simulink model "CiEngineCore"  (R2020a)
settings: Solver=VariableStepAuto  StartTime=0.0  StopTime=inf  RelTol=1e-3  EnableMultiTasking=on
model workspace (MAT data in the model file):
  AirFilterArea = 0.000962112750162
  AirIntakeVol = 0.0018
  C_eng = 40000
  CompEff = [0.2 0.2 0.2 0.2 0.2 0.2 0.2 0.2 0.2 0.2 0.2 0.2 ... (6000 elements, 60x100)]
  CompMassFlwRate = [0 0.00256701884694 0.00511455880808 0.00766649491749 0.0102195028494 0.0127729401774 0.0153265889731 0.017880362476 0.0204342099213 0.0229881081418 0.0255420430633 0.0280960028754 ... (6000 elements, 60x100)]
  CompPrsRatioBreakPoints = [1 1.02808080808 1.05616161616 1.08424242424 1.11232323232 1.1404040404 1.16848484848 1.19656565657 1.22464646465 1.25272727273 1.28080808081 1.30888888889 1.33696969697 1.36505050505 1.39313131313 1.42121212121 1.44929292929 1.47737373737 1.50545454545 1.53353535354 1.56161616162 1.5896969697 1.61777777778 1.64585858586 1.67393939394 1.70202020202 1.7301010101 1.75818181818 1.78626262626 1.81434343434 1.84242424242 1.87050505051 1.89858585859 1.92666666667 1.95474747475 1.98282828283 2.01090909091 2.03898989899 2.06707070707 2.09515151515 2.12323232323 2.15131313131 2.17939393939 2.20747474747 2.23555555556 2.26363636364 2.29171717172 2.3197979798 2.34787878788 2.37595959596 2.40404040404 2.43212121212 2.4602020202 2.48828282828 2.51636363636 2.54444444444 2.57252525253 2.60060606061 2.62868686869 2.65676767677 2.68484848485 2.71292929293 2.74101010101 2.76909090909 2.79717171717 2.82525252525 2.85333333333 2.88141414141 2.90949494949 2.93757575758 2.96565656566 2.99373737374 3.02181818182 3.0498989899 3.07797979798 3.10606060606 3.13414141414 3.16222222222 3.1903030303 3.21838383838 3.24646464646 3.27454545455 3.30262626263 3.33070707071 3.35878787879 3.38686868687 3.41494949495 3.44303030303 3.47111111111 3.49919191919 3.52727272727 3.55535353535 3.58343434343 3.61151515152 3.6395959596 3.66767676768 3.69575757576 3.72383838384 3.75191919192 3.78]
  CompRefPrs = 101325
  CompRefTemp = 300
  CompSpdBreakPoints = [0 422.344846438 844.689692876 1267.03447648 1689.3794067 2111.72412747 2534.06895296 2956.4139879 3378.75881339 3801.10374361 4223.44825494 4645.79349931 5068.13790593 5490.48294086 5912.8279758 6335.17238241 6757.51762678 7179.86182396 7602.20748721 8024.55231271 8446.89650988 8869.24133538 9291.58699863 9713.9311958 10136.2759166 10558.6216845 10980.9658817 11403.3100789 11825.6558469 12248.0005676 12670.3447648 13092.6904281 13515.0352536 13937.3794507 14359.7246951 14782.0688923 15204.4151839 15626.759381 16049.1046254 16471.4488226 16893.7930198 17316.1382641 17738.4824613 18160.8287529 18583.1729501 19005.5181944 19427.8623916 19850.207636 20272.5518332 20694.8981247 21117.2423219 21539.5865191 21961.9317635 22384.2770078 22806.621205 23228.9654022 23651.3116937 24073.6558909 24496.0011353 24918.3453325]
  CoolantTemp = 310
  Cps = 2
  EgrArea = 0.000314159265359
  EgrCoolantTemp = 360
  EgrEffectiveness = 0.8
  ExhSysArea = 0.000804247719319
  ExhSysVol = 0.0008
  IcEffectiveness = 0.9
  LHV = 47300000
  NCyl = 4
  Pstd = 101325
  Rair = 287.05
  Rexh = 297
  Sinj = 6.45161290323
  T_cool_start = 355
  T_coolnt_init = 355
  T_coolnt_max = 375
  Tstd = 293.15
  TurbEff = [0.008 0.008 0.008 0.008 0.008 0.008 0.008 0.008 0.008 0.008 0.008 0.008 ... (28800 elements, 60x80x6)]
  TurbMassFlwRate = [0 0 0 0 0 0 0 0 0 0 0 0 ... (28800 elements, 60x80x6)]
  TurbPrsRatioBreakPoints = [1 1.03481012658 1.06962025316 1.10443037975 1.13924050633 1.17405063291 1.20886075949 1.24367088608 1.27848101266 1.31329113924 1.34810126582 1.38291139241 1.41772151899 1.45253164557 1.48734177215 1.52215189873 1.55696202532 1.5917721519 1.62658227848 1.66139240506 1.69620253165 1.73101265823 1.76582278481 1.80063291139 1.83544303797 1.87025316456 1.90506329114 1.93987341772 1.9746835443 2.00949367089 2.04430379747 2.07911392405 2.11392405063 2.14873417722 2.1835443038 2.21835443038 2.25316455696 2.28797468354 2.32278481013 2.35759493671 2.39240506329 2.42721518987 2.46202531646 2.49683544304 2.53164556962 2.5664556962 2.60126582278 2.63607594937 2.67088607595 2.70569620253 2.74050632911 2.7753164557 2.81012658228 2.84493670886 2.87974683544 2.91455696203 2.94936708861 2.98417721519 3.01898734177 3.05379746835 3.08860759494 3.12341772152 3.1582278481 3.19303797468 3.22784810127 3.26265822785 3.29746835443 3.33227848101 3.36708860759 3.40189873418 3.43670886076 3.47151898734 3.50632911392 3.54113924051 3.57594936709 3.61075949367 3.64556962025 3.68037974684 3.71518987342 3.75]
  TurbRackBreakPoints = [0 0.2 0.3 0.5 0.7 1]
  TurbRefPrs = 101325
  TurbRefTemp = 300
  TurbSpdBreakPoints = [0 267.361773363 534.723546727 802.08532009 1069.44709345 1336.80886682 1604.17064018 1871.53241354 2138.89418691 2406.25596027 2673.61773363 2940.979507 3208.34128036 3475.70305372 3743.06482709 4010.42660045 4277.78837381 4545.15014718 4812.51192054 5079.8736939 5347.23546727 5614.59724063 5881.95901399 6149.32078736 6416.68256072 6684.04433408 6951.40610745 7218.76788081 7486.12965417 7753.49142754 8020.8532009 8288.21497426 8555.57674763 8822.93852099 9090.30029435 9357.66206772 9625.02384108 9892.38561444 10159.7473878 10427.1091612 10694.4709345 10961.8327079 11229.1944813 11496.5562546 11763.918028 12031.2798014 12298.6415747 12566.0033481 12833.3651214 13100.7268948 13368.0886682 13635.4504415 13902.8122149 14170.1739883 14437.5357616 14704.897535 14972.2593083 15239.6210817 15506.9828551 15774.3446284]
  TurboInertia = 6e-06
  Vd = 0.0015
  Vexh = 0.000696349540849
  Vint = 0.00286
  afr_stoich = 14.6
  cp_air = 1005
  cp_exh = 1005
  f_co = [1.40212981041e-06 1.40212981041e-06 1.6332261526e-06 1.85316257772e-06 2.13933731744e-06 2.5578774362e-06 3.5801963158e-06 5.71066968323e-06 9.06691784867e-06 1.17856264254e-05 1.13266430068e-05 1.17075290539e-05 ... (240 elements, 16x15)]
  f_co2 = [0.0565058276487 0.0565058276487 0.0680775298139 0.0795416117649 0.0927502758383 0.108898516704 0.135970777083 0.163224038089 0.18390566243 0.187824483941 0.180854201863 0.181624048607 ... (240 elements, 16x15)]
  f_exhfrac_n_bpt = [750 1053.57142857 1357.14285714 1660.71428571 1964.28571429 2267.85714286 2571.42857143 2875 3178.57142857 3482.14285714 3785.71428571 4089.28571429 4392.85714286 4696.42857143 5000]
  f_exhfrac_trq_bpt = [0 15 26.4285714286 37.8571428571 49.2857142857 60.7142857143 72.1428571429 83.5714285714 95 106.428571429 117.857142857 129.285714286 140.714285714 152.142857143 163.571428571 175]
  f_fric_temp_bpt = [274 276 278 280 282 284 286 288 290 292 294 296 298 300 302 304 306 308 310 312 314 316 318 320 322 324 326 328 330 332 334 336 338 340 342 344 346 348 350 352 354 356 358 360 362 364 366 368 370 372 374 376 378 380]
  f_fric_temp_mod = [3.96 3.22 2.56 2.26 2.11 2 1.9 1.83 1.76 1.7 1.65 1.6 1.55 1.49 1.44 1.41 1.38 1.35 1.32 1.3 1.27 1.25 1.24 1.21 1.2 1.18 1.16 1.15 1.13 1.12 1.11 1.1 1.09 1.08 1.07 1.06 1.05 1.05 1.04 1.03 1.02 1.02 1.01 1.01 1 1 1 0.999 0.997 0.995 0.993 0.991 0.989 0.987]
  f_hc = [1.08896576916e-07 1.08896576916e-07 1.53414498342e-07 2.00715453959e-07 2.48790869997e-07 2.97869368014e-07 3.52504999231e-07 4.04349945817e-07 4.52780325277e-07 4.91342452993e-07 4.91996758973e-07 4.96487624267e-07 ... (240 elements, 16x15)]
  f_nox = [9.38886565825e-05 9.38886565825e-05 0.000158278744526 0.000381657424268 0.00062836202089 0.000865097048745 0.000965103000667 0.00083216127124 0.00082959112316 0.00143554359074 0.00196340813932 0.0020351396325 ... (240 elements, 16x15)]
  f_nv = [0.954646224834 0.927678310575 0.901063682417 0.875710037198 0.852450535311 0.831986822876 0.814844392337 0.80134438932 0.791593989181 0.785495277781 0.782770492696 0.782999798686 ... (450 elements, 30x15)]
  f_nv_n_bpt = [1000 1285.71428571 1571.42857143 1857.14285714 2142.85714286 2428.57142857 2714.28571429 3000 3285.71428571 3571.42857143 3857.14285714 4142.85714286 4428.57142857 4714.28571429 5000]
  f_nv_prs_bpt = [95 100.344827586 105.689655172 111.034482759 116.379310345 121.724137931 127.068965517 132.413793103 137.75862069 143.103448276 148.448275862 153.793103448 159.137931034 164.482758621 169.827586207 175.172413793 180.517241379 185.862068966 191.206896552 196.551724138 201.896551724 207.24137931 212.586206897 217.931034483 223.275862069 228.620689655 233.965517241 239.310344828 244.655172414 250]
  f_t_exh = [358.711368346 429.963145924 497.987869771 559.016510887 625.497016294 690.207854611 731.780908025 749.899407528 764.155922317 789.797182974 824.513264157 858.92580636 ... (240 elements, 16x15)]
  f_t_exh_f_bpt = [0 3.57 6.855 10.14 13.425 16.71 19.995 23.28 26.565 29.85 33.135 36.42 39.705 42.99 46.275 49.56]
  f_t_exh_n_bpt = [1000 1285.71428571 1571.42857143 1857.14285714 2142.85714286 2428.57142857 2714.28571429 3000 3285.71428571 3571.42857143 3857.14285714 4142.85714286 4428.57142857 4714.28571429 5000]
  f_tq_nf = [0 4.01032735147 17.4541547029 30.8399626872 43.6894710619 54.6724182266 65.9817429981 74.8844587697 82.0625281792 91.0474591726 100.604737295 107.761633858 ... (320 elements, 20x16)]
  f_tq_nf_f_bpt = [0 2.63157894737 5.26315789474 7.89473684211 10.5263157895 13.1578947368 15.7894736842 18.4210526316 21.0526315789 23.6842105263 26.3157894737 28.9473684211 31.5789473684 34.2105263158 36.8421052632 39.4736842105 42.1052631579 44.7368421053 47.3684210526 50]
  f_tq_nf_n_bpt = [0 1000 1285.71428571 1571.42857143 1857.14285714 2142.85714286 2428.57142857 2714.28571429 3000 3285.71428571 3571.42857143 3857.14285714 4142.85714286 4428.57142857 4714.28571429 5000]
  f_tqs_emap = [101325 101325 101325 101325 101325 101325 101325 101325 101325 101325 101325 101325 ... (240 elements, 15x16)]
  f_tqs_exht = [293.15 293.15 293.15 293.15 293.15 293.15 293.15 293.15 293.15 293.15 293.15 293.15 ... (240 elements, 15x16)]
  f_tqs_exht_fuelpress_eff = [1  1  1  1  1  1  1  1  1  1  1  1  1  1  1  1; 1  1  1  1  1  1  1  1  1  1  1  1  1  1  1  1; 1  1  1  1  1  1  1  1  1  1  1  1  1  1  1  1; 1  1  1  1  1  1  1  1  1  1  1  1  1  1  1  1; 1  1  1  1  1  1  1  1  1  1  1  1  1  1  1  1; 1  1  1  1  1  1  1  1  1  1  1  1  1  1  1  1; 1  1  1  1  1  1  1  1  1  1  1  1  1  1  1  1; 1  1  1  1  1  1  1  1  1  1  1  1  1  1  1  1; 1  1  1  1  1  1  1  1  1  1  1  1  1  1  1  1; 1  1  1  1  1  1  1  1  1  1  1  1  1  1  1  1; 1  1  1  1  1  1  1  1  1  1  1  1  1  1  1  1; 1  1  1  1  1  1  1  1  1  1  1  1  1  1  1  1; 1  1  1  1  1  1  1  1  1  1  1  1  1  1  1  1; 1  1  1  1  1  1  1  1  1  1  1  1  1  1  1  1; 1  1  1  1  1  1  1  1  1  1  1  1  1  1  1  1]
  f_tqs_exht_mainsoi_eff = [1 1 1 1 1 1 1 1 1 1 1 1 ... (240 elements, 15x16)]
  f_tqs_exht_map_eff = [1.11693337379 1.10383565741 1.07527138779 1.03804427558 1 0.975297725101 0.950398019177 0.924393698482 0.899021655666 0.876045599233 0.858573316119 0.844444824038 ... (225 elements, 15x15)]
  f_tqs_exht_mat_eff = [1 1 1 1 1 1 1 1 1 1 1 1 ... (240 elements, 15x16)]
  f_tqs_exht_o2pct_eff = [1 1 1 1 1 1 1 1 1 1 1 1 ... (240 elements, 15x16)]
  f_tqs_exht_post_inj_wall_htc = 0
  f_tqs_f_bpt = [0; 3.57142857143; 7.14285714286; 10.7142857143; 14.2857142857; 17.8571428571; 21.4285714286; 25; 28.5714285714; 32.1428571429; 35.7142857143; 39.2857142857; 42.8571428571; 46.4285714286; 50]
  f_tqs_f_burned_soi_limit = 500
  f_tqs_f_inj_type = 0
  f_tqs_f_post_sum_bpt = [0 3.57142857143 7.14285714286 10.7142857143 14.2857142857 17.8571428571 21.4285714286 25 28.5714285714 32.1428571429 35.7142857143 39.2857142857 42.8571428571 46.4285714286 50]
  f_tqs_fmep = [0 0 0 0 0 0 0 0 0 0 0 0 ... (240 elements, 15x16)]
  f_tqs_fric_temp_bpt = [273.15; 275.166037736; 277.182075472; 279.198113208; 281.214150943; 283.230188679; 285.246226415; 287.262264151; 289.278301887; 291.294339623; 293.310377358; 295.326415094; 297.34245283; 299.358490566; 301.374528302; 303.390566038; 305.406603774; 307.422641509; 309.438679245; 311.454716981; 313.470754717; 315.486792453; 317.502830189; 319.518867925; 321.53490566; 323.550943396; 325.566981132; 327.583018868; 329.599056604; 331.61509434; 333.631132075; 335.647169811; 337.663207547; 339.679245283; 341.695283019; 343.711320755; 345.727358491; 347.743396226; 349.759433962; 351.775471698; 353.791509434; 355.80754717; 357.823584906; 359.839622642; 361.855660377; 363.871698113; 365.887735849; 367.903773585; 369.919811321; 371.935849057; 373.951886792; 375.967924528; 377.983962264; 380]
  f_tqs_fric_temp_mod = [1 1 1 1 1 1 1 1 1 1 1 1 ... (864 elements, 54x16)]
  f_tqs_fuelpress = [100  100  100  100  100  100  100  100  100  100  100  100  100  100  100  100; 100  100  100  100  100  100  100  100  100  100  100  100  100  100  100  100; 100  100  100  100  100  100  100  100  100  100  100  100  100  100  100  100; 100  100  100  100  100  100  100  100  100  100  100  100  100  100  100  100; 100  100  100  100  100  100  100  100  100  100  100  100  100  100  100  100; 100  100  100  100  100  100  100  100  100  100  100  100  100  100  100  100; 100  100  100  100  100  100  100  100  100  100  100  100  100  100  100  100; 100  100  100  100  100  100  100  100  100  100  100  100  100  100  100  100; 100  100  100  100  100  100  100  100  100  100  100  100  100  100  100  100; 100  100  100  100  100  100  100  100  100  100  100  100  100  100  100  100; 100  100  100  100  100  100  100  100  100  100  100  100  100  100  100  100; 100  100  100  100  100  100  100  100  100  100  100  100  100  100  100  100; 100  100  100  100  100  100  100  100  100  100  100  100  100  100  100  100; 100  100  100  100  100  100  100  100  100  100  100  100  100  100  100  100; 100  100  100  100  100  100  100  100  100  100  100  100  100  100  100  100]
  f_tqs_fuelpress_delta_bpt = [-30; -25.7142857143; -21.4285714286; -17.1428571429; -12.8571428571; -8.57142857143; -4.28571428571; 0; 4.28571428571; 8.57142857143; 12.8571428571; 17.1428571429; 21.4285714286; 25.7142857143; 30]
  f_tqs_fuelpress_eff = [1  1  1  1  1  1  1  1  1  1  1  1  1  1  1  1; 1  1  1  1  1  1  1  1  1  1  1  1  1  1  1  1; 1  1  1  1  1  1  1  1  1  1  1  1  1  1  1  1; 1  1  1  1  1  1  1  1  1  1  1  1  1  1  1  1; 1  1  1  1  1  1  1  1  1  1  1  1  1  1  1  1; 1  1  1  1  1  1  1  1  1  1  1  1  1  1  1  1; 1  1  1  1  1  1  1  1  1  1  1  1  1  1  1  1; 1  1  1  1  1  1  1  1  1  1  1  1  1  1  1  1; 1  1  1  1  1  1  1  1  1  1  1  1  1  1  1  1; 1  1  1  1  1  1  1  1  1  1  1  1  1  1  1  1; 1  1  1  1  1  1  1  1  1  1  1  1  1  1  1  1; 1  1  1  1  1  1  1  1  1  1  1  1  1  1  1  1; 1  1  1  1  1  1  1  1  1  1  1  1  1  1  1  1; 1  1  1  1  1  1  1  1  1  1  1  1  1  1  1  1; 1  1  1  1  1  1  1  1  1  1  1  1  1  1  1  1]
  f_tqs_imep_post_corr = [0  0  0  0  0  0  0  0  0  0  0  0  0  0  0; 0  0  0  0  0  0  0  0  0  0  0  0  0  0  0; 0  0  0  0  0  0  0  0  0  0  0  0  0  0  0; 0  0  0  0  0  0  0  0  0  0  0  0  0  0  0; 0  0  0  0  0  0  0  0  0  0  0  0  0  0  0; 0  0  0  0  0  0  0  0  0  0  0  0  0  0  0; 0  0  0  0  0  0  0  0  0  0  0  0  0  0  0; 0  0  0  0  0  0  0  0  0  0  0  0  0  0  0; 0  0  0  0  0  0  0  0  0  0  0  0  0  0  0; 0  0  0  0  0  0  0  0  0  0  0  0  0  0  0; 0  0  0  0  0  0  0  0  0  0  0  0  0  0  0; 0  0  0  0  0  0  0  0  0  0  0  0  0  0  0; 0  0  0  0  0  0  0  0  0  0  0  0  0  0  0; 0  0  0  0  0  0  0  0  0  0  0  0  0  0  0; 0  0  0  0  0  0  0  0  0  0  0  0  0  0  0]
  f_tqs_imepg = [0 158686.534722 343074.265588 507983.203346 653190.552872 792520.266872 898623.174707 1024926.34814 1192408.65419 1362289.29874 1538616.81914 1722468.1753 ... (240 elements, 15x16)]
  f_tqs_lambda_bpt = [1.5 1.67857142857 1.85714285714 2.03571428571 2.21428571429 2.39285714286 2.57142857143 2.75 2.92857142857 3.10714285714 3.28571428571 3.46428571429 3.64285714286 3.82142857143 4]
  f_tqs_mainsoi = [-5.65203706782 -5.56485950617 -5.32737749535 -4.90693102774 -4.39157989496 -2.6685350622 -1.13269707429 -0.442811837066 0.0846384555918 0.793458776955 1.62426195607 2.45698560821 ... (240 elements, 15x16)]
  f_tqs_mainsoi_delta_bpt = [-15; -12.8571428571; -10.7142857143; -8.57142857143; -6.42857142857; -4.28571428571; -2.14285714286; 0; 2.14285714286; 4.28571428571; 6.42857142857; 8.57142857143; 10.7142857143; 12.8571428571; 15]
  f_tqs_mainsoi_eff = [1 1 1 1 1 1 1 1 1 1 1 1 ... (240 elements, 15x16)]
  f_tqs_map = [101325 101325 101325 101325 101325 101325 101325 101325 101325 101325 101325 101325 ... (240 elements, 15x16)]
  f_tqs_map_eff = [0.876486797315 0.914614445767 0.94792295911 0.975703338034 1 1.02743787204 1.05216674291 1.07395048632 1.09371107566 1.11066007626 1.12521245816 1.14202789912 ... (225 elements, 15x15)]
  f_tqs_map_ratio_bpt = [0.8; 0.85; 0.9; 0.95; 1; 1.05; 1.1; 1.15; 1.2; 1.25; 1.3; 1.35; 1.4; 1.45; 1.5]
  f_tqs_mat = [293.15 293.15 293.15 293.15 293.15 293.15 293.15 293.15 293.15 293.15 293.15 293.15 ... (240 elements, 15x16)]
  f_tqs_mat_delta_bpt = [-55; -50; -45; -40; -35; -30; -25; -20; -15; -10; -5; 0; 5; 10; 15]
  f_tqs_mat_eff = [1 1 1 1 1 1 1 1 1 1 1 1 ... (240 elements, 15x16)]
  f_tqs_n_bpt = [0 500 750 1000 1250 1500 1750 2000 2250 2500 2750 3000 3250 3500 3750 4000]
  f_tqs_o2pct = [18.6138636402 19.5619833676 20.7378306586 22.1536730517 23.4120452691 23.8418651452 23.8693762547 23.8866954757 24.0193105899 24.2672589018 24.5893674985 24.9537951111 ... (240 elements, 15x16)]
  f_tqs_o2pct_delta_bpt = [-2; -1.33333333333; -0.666666666667; 0; 0.666666666667; 1.33333333333; 2; 2.66666666667; 3.33333333333; 4; 4.66666666667; 5.33333333333; 6; 6.66666666667; 7.33333333333]
  f_tqs_o2pct_eff = [1 1 1 1 1 1 1 1 1 1 1 1 ... (240 elements, 15x16)]
  f_tqs_pmep = [0 0 0 0 0 0 0 0 0 0 0 0 ... (240 elements, 15x16)]
  f_tqs_soi_post_cent_bpt = [150 160.714285714 171.428571429 182.142857143 192.857142857 203.571428571 214.285714286 225 235.714285714 246.428571429 257.142857143 267.857142857 278.571428571 289.285714286 300]
  fuel_lhv = 42000000
  tau_cool = 3000
undefined symbols (not defined in the file or in its folder): ThrAngToC
libraries: autolibfundflw x11, autolibboost x3, autolibcoreeng x1, simulink x1
(part 1 of 2)
settings Model: ModifiedByFormat=The MathWorks, Inc.  OrderedModelArguments=off  Creator=The MathWorks, Inc.  LastModifiedBy=The MathWorks, Inc.
settings SolverCC: DecoupledContinuousIntegration=on
settings DataIOCC: DSMLogging=off  ReturnWorkspaceOutputs=off
settings DebuggingCC: PregeneratedLibrarySubsystemCodeDiagnostic=none  ArithmeticOperatorsInVariantConditions=warning
settings SFSimCC: SimUseLocalCustomCode=off  CustomCodeUndefinedFunction=UseInterfaceOnly
settings RTWCC: RTWUseLocalCustomCode=off
settings CodeAppCC: StateflowObjectComments=on
settings GRTTargetCC: TargetLangStandard=C89/C90 (ANSI)
settings ConfigComp: CovMetricSettings=dsw  CovHtmlReporting=on  CovSaveCumulativeToWorkspaceVar=on  CovSaveSingleToWorkspaceVar=on  CovShowResultsExplorer=off  CovExternalEMLEnable=off
settings SimscapeCC: SimscapeNormalizeSystem=off  SimscapeNominalValues={1, 'bar'; 1, 'cm^3/s'; 1, 'bar*kg/s'; 1, 'kJ/kg'; 1, 'kW'; }

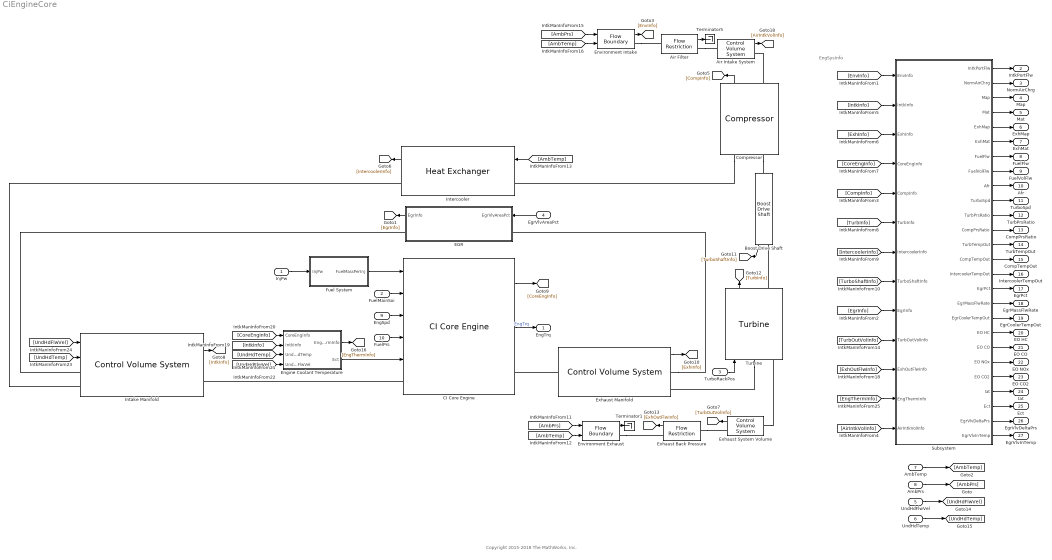
== system CiEngineCore ==
  note: EngSysInfo
  note: Copyright 2015-2018 The MathWorks, Inc.
  InjPw : Inport
  FuelMainSoi : Inport  Port=2
  TurboRackPos : Inport  Port=3
  EgrVlvAreaPct : Inport  Port=4
  UndHdFlwVel : Inport  Port=5
  UndHdTemp : Inport  Port=6
  AmbTemp : Inport  Port=7
  AmbPrs : Inport  Port=8
  EngSpd : Inport  Port=9
  FuelPrs : Inport  Port=10
  Air Filter : autolibfundflw/Flow Restriction  AreaPopup=Constant  ImageTypePopup=Cold  gamma=cp_air/(cp_air-Rair)  R=Rair  Plim=0.99  Aorf_cnst=AirFilterArea  Cd_cnst=1  Cd_ext=1  Dthr=50  ThrCd=[0.001; 0.735]  ThrAngBpts=[0; 90]
      settings: SourceProductBaseCode=PW
  Air Intake System : autolibfundflw/Control Volume System  NumInletPorts=1  NumOutletPorts=1  HeatTransferModelPopup=Constant  ImageTypePopup=Cold  Vch=AirIntakeVol  Pinit=101325  Tinit=298  R=Rair  cp=cp_air  q_he=0  ext_tbl=[40 160 740 2000]  ext_bpts=linspace(0,180,4)  Aext_conv=0.125  m_wall=7  cp_wall=900  Tmass=293.15  Dext_cond=0.004  Aext_cond=0.003  kext=25  Dint_cond=0.004  Aint_cond=0.003  kint=25  int_tbl=[40 160 740 2000]  int_bpts=linspace(0.0020,0.1100,4)  Aint_conv=0.125
      settings: SourceProductBaseCode=PW
  Boost Drive Shaft : autolibboost/Boost Drive Shaft  ShaftConfigPopup=Turbocharger  AddTrqTypePopup=No external torque  J_shaft=TurboInertia  w_0=0.0001  w_min=0.0001  w_max=1e6  eta_mech=1
      settings: SourceProductBaseCode=PW
  CI Core Engine : autolibcoreeng/CI Core Engine  TrqOptionPopup=Torque Structure  NCyl=NCyl  Tstd=Tstd  Cps=Cps  Vd=Vd  Rair=Rair  Pstd=Pstd  f_nv=f_nv  f_nv_prs_bpt=f_nv_prs_bpt  f_nv_n_bpt=f_nv_n_bpt  f_tq_nf=f_tq_nf  f_tq_nf_f_bpt=f_tq_nf_f_bpt  f_tq_nf_n_bpt=f_tq_nf_n_bpt  f_tqs_f_bpt=f_tqs_f_bpt  f_tqs_n_bpt=f_tqs_n_bpt  f_tqs_mainsoi=f_tqs_mainsoi  f_tqs_map=f_tqs_map  f_tqs_emap=f_tqs_emap  f_tqs_mat=f_tqs_mat  f_tqs_o2pct=f_tqs_o2pct  f_tqs_fuelpress=f_tqs_fuelpress  f_tqs_imepg=f_tqs_imepg  f_tqs_fmep=f_tqs_fmep  f_tqs_pmep=f_tqs_pmep  f_tqs_fric_temp_mod=f_tqs_fric_temp_mod  f_tqs_fric_temp_bpt=f_tqs_fric_temp_bpt  f_tqs_mainsoi_eff=f_tqs_mainsoi_eff  f_tqs_mainsoi_delta_bpt=f_tqs_mainsoi_delta_bpt  f_tqs_map_eff=f_tqs_map_eff  f_tqs_map_ratio_bpt=f_tqs_map_ratio_bpt  f_tqs_lambda_bpt=f_tqs_lambda_bpt  f_tqs_mat_eff=f_tqs_mat_eff  f_tqs_mat_delta_bpt=f_tqs_mat_delta_bpt  f_tqs_o2pct_eff=f_tqs_o2pct_eff  f_tqs_o2pct_delta_bpt=f_tqs_o2pct_delta_bpt  f_tqs_fuelpress_eff=f_tqs_fuelpress_eff  f_tqs_fuelpress_delta_bpt=f_tqs_fuelpress_delta_bpt  f_tqs_f_inj_type=f_tqs_f_inj_type  f_tqs_imep_post_corr=f_tqs_imep_post_corr  f_tqs_f_post_sum_bpt=f_tqs_f_post_sum_bpt  f_tqs_soi_post_cent_bpt=f_tqs_soi_post_cent_bpt  f_tqs_f_burned_soi_limit=f_tqs_f_burned_soi_limit  f_t_exh=f_t_exh  f_t_exh_f_bpt=f_t_exh_f_bpt  f_t_exh_n_bpt=f_t_exh_n_bpt  f_tqs_exht=f_tqs_exht  f_tqs_exht_mainsoi_eff=f_tqs_exht_mainsoi_eff  f_tqs_exht_map_eff=f_tqs_exht_map_eff  f_tqs_exht_mat_eff=f_tqs_exht_mat_eff  f_tqs_exht_o2pct_eff=f_tqs_exht_o2pct_eff  f_tqs_exht_fuelpress_eff=f_tqs_exht_fuelpress_eff  f_tqs_exht_post_inj_wall_htc=f_tqs_exht_post_inj_wall_htc  CO2EmissionsCheckbox=on  COEmissionsCheckbox=on  NOxEmissionsCheckbox=on  HCEmissionsCheckbox=on  PMEmissionsCheckbox=off  f_CO2_frac=f_co2  f_CO_frac=f_co  f_HC_frac=f_hc  f_NOx_frac=f_nox  f_PM_frac=[0 0 0 0 0 0 0 0 0 0 0 0 0 0 0;0 0 0 0 0 0 0 0 0 0 0 0 0 0 0;0 0 0 0 0 0 0 0 0 0 0 0 0 0 0;0 0 0 0 0 0 0 0 0 0 0 0 0 0 0;0 0 0 0 0 0 0 0 0 0 0 0 0 0 0;0 0 0 0 0 0 0 0 0 0 0 0 0 0 0;0 0 0 0 0 0 0 0 0 0 0 0 0 0 0;0 0 0 0 0 0 0 0 0 0 0 0 0 0 0;0 0 0 0 0 0 0 0 0 0 0 0 0 0 0;0 0 0 0 0 0 0 0 0 0 0 0 0 0 0;0 0 0 0 0 0 0 0 0 0 0 0 0 0 0;0 0 0 0 0 0 0 0 0 0 0 0 0 0 0;0 0 0 0 0 0 0 0 0 0 0 0 0 0 0;0 0 0 0 0 0 0 0 0 0 0 0 0 0 0;0 0 0 0 0 0 0 0 0 0 0 0 0 0 0;0 0 0 0 0 0 0 0 0 0 0 0 0 0 0]  f_exhfrac_n_bpt=f_exhfrac_n_bpt  f_exhfrac_trq_bpt=f_exhfrac_trq_bpt  cp_exh=cp_exh  afr_stoich=afr_stoich  fuel_lhv=fuel_lhv  fuel_sg=0.832
      settings: SourceProductBaseCode=PW
  Compressor : autolibboost/Compressor  mdot_corr_tbl=CompMassFlwRate  eta_comp_tbl=CompEff  w_corr_bpts1=CompSpdBreakPoints  Pr_bpts2=CompPrsRatioBreakPoints  T_ref=CompRefTemp  P_ref=CompRefPrs  R=Rair  cp=cp_air  CalCmprsData={'', '', 'MassFlwRate', 'Eff'}
      settings: SourceProductBaseCode=PW
  EGR : Subsystem
  Engine Coolant Temperature : Subsystem
  Environment Exhaust : autolibfundflw/Flow Boundary  PrsTempSrcPopup=External input  ImageTypePopup=Hot  Pcnst=101325  Tcnst=298.15  cp=cp_air
      settings: SourceProductBaseCode=PW
  Environment Intake : autolibfundflw/Flow Boundary  PrsTempSrcPopup=External input  ImageTypePopup=Cold  Pcnst=101325  Tcnst=298.15  cp=cp_air
      settings: SourceProductBaseCode=PW
  Exhaust Back Pressure : autolibfundflw/Flow Restriction  AreaPopup=Constant  ImageTypePopup=Hot  gamma=cp_exh/(cp_exh-Rexh)  R=Rexh  Plim=0.99  Aorf_cnst=ExhSysArea  Cd_cnst=1  Cd_ext=1  Dthr=50  ThrCd=[0.001; 0.735]  ThrAngBpts=[0; 90]
      settings: SourceProductBaseCode=PW
  Exhaust Manifold : autolibfundflw/Control Volume System  NumInletPorts=1  NumOutletPorts=2  HeatTransferModelPopup=Constant  ImageTypePopup=Hot  Vch=Vexh  Pinit=101325  Tinit=298  R=Rexh  cp=cp_exh  q_he=0  ext_tbl=[40 160 740 2000]  ext_bpts=linspace(0,180,4)  Aext_conv=0.125  m_wall=7  cp_wall=900  Tmass=293.15  Dext_cond=0.004  Aext_cond=0.003  kext=25  Dint_cond=0.004  Aint_cond=0.003  kint=25  int_tbl=[40 160 740 2000]  int_bpts=linspace(0.0020,0.1100,4)  Aint_conv=0.125
      settings: SourceProductBaseCode=PW
  Exhaust System Volume : autolibfundflw/Control Volume System  NumInletPorts=1  NumOutletPorts=1  HeatTransferModelPopup=Constant  ImageTypePopup=Hot  Vch=ExhSysVol  Pinit=101325  Tinit=298  R=Rexh  cp=cp_exh  q_he=0  ext_tbl=[40 160 740 2000]  ext_bpts=linspace(0,180,4)  Aext_conv=0.125  m_wall=7  cp_wall=900  Tmass=293.15  Dext_cond=0.004  Aext_cond=0.003  kext=25  Dint_cond=0.004  Aint_cond=0.003  kint=25  int_tbl=[40 160 740 2000]  int_bpts=linspace(0.0020,0.1100,4)  Aint_conv=0.125
      settings: SourceProductBaseCode=PW
  Fuel System : Subsystem
  Intake Manifold : autolibfundflw/Control Volume System  NumInletPorts=2  NumOutletPorts=1  HeatTransferModelPopup=External wall convection  ImageTypePopup=Cold  Vch=Vint  Pinit=101325  Tinit=298  R=Rair  cp=cp_air  q_he=0  ext_tbl=[40 160 740 2000]  ext_bpts=linspace(0,180,4)  Aext_conv=0.125  m_wall=7  cp_wall=900  Tmass=293.15  Dext_cond=0.004  Aext_cond=0.003  kext=25  Dint_cond=0.004  Aint_cond=0.003  kint=25  int_tbl=[40 160 740 2000]  int_bpts=linspace(0.0020,0.1100,4)  Aint_conv=0.125
      settings: SourceProductBaseCode=PW
  Intercooler : autolibfundflw/Heat Exchanger  EffctModelPopup=Constant  CoolTempInputPopup=External input  ImageTypePopup=Intercooler  ep_cnst=IcEffectiveness  T_cool_cnst=CoolantTemp  cp=cp_air
      settings: SourceProductBaseCode=PW
  Subsystem : Subsystem
  Terminator1 : Terminator
  Terminator5 : Terminator
  Turbine : autolibboost/Turbine  TurbTypePopup=Variable geometry  WgIncludeCheckbox=off  mdot_corrfx_tbl=TurbMassFlwRate  mdot_corrvr_tbl=TurbMassFlwRate  eta_turbfx_tbl=TurbEff  eta_turbvr_tbl=TurbEff  w_corrfx_bpts1=TurbSpdBreakPoints  w_corrvr_bpts2=TurbSpdBreakPoints  Pr_fx_bpts2=TurbPrsRatioBreakPoints  Pr_vr_bpts2=TurbPrsRatioBreakPoints  L_rack_bpts3=TurbRackBreakPoints  T_ref=TurbRefTemp  P_ref=TurbRefPrs  mdot_thresh=1e-6  A_wgopen=WgArea  Plim_wg=.99  R=Rexh  cp=cp_exh  CalFixedMapsData={'', '', 'FixedTurbine'}  CalVgtMapsData={'', '', 'Vgt-Point-by-Point'}
      settings: SourceProductBaseCode=PW
  EngTrq : Outport  VectorParamsAs1DForOutWhenUnconnected=off
  IntkPortFlw : Outport  Port=2  VectorParamsAs1DForOutWhenUnconnected=off
  NormAirChrg : Outport  Port=3  VectorParamsAs1DForOutWhenUnconnected=off
  Map : Outport  Port=4  VectorParamsAs1DForOutWhenUnconnected=off
  Mat : Outport  Port=5  VectorParamsAs1DForOutWhenUnconnected=off
  ExhMap : Outport  Port=6  VectorParamsAs1DForOutWhenUnconnected=off
  ExhMat : Outport  Port=7  VectorParamsAs1DForOutWhenUnconnected=off
  FuelFlw : Outport  Port=8  VectorParamsAs1DForOutWhenUnconnected=off
  FuelVolFlw : Outport  Port=9  VectorParamsAs1DForOutWhenUnconnected=off
  Afr : Outport  Port=10  VectorParamsAs1DForOutWhenUnconnected=off
  TurboSpd : Outport  Port=11  VectorParamsAs1DForOutWhenUnconnected=off
  TurbPrsRatio : Outport  Port=12  VectorParamsAs1DForOutWhenUnconnected=off
  CompPrsRatio : Outport  Port=13  VectorParamsAs1DForOutWhenUnconnected=off
  TurbTempOut : Outport  Port=14  VectorParamsAs1DForOutWhenUnconnected=off
  CompTempOut : Outport  Port=15  VectorParamsAs1DForOutWhenUnconnected=off
  IntercoolerTempOut : Outport  Port=16  VectorParamsAs1DForOutWhenUnconnected=off
  EgrPct : Outport  Port=17  VectorParamsAs1DForOutWhenUnconnected=off
  EgrMassFlwRate : Outport  Port=18  VectorParamsAs1DForOutWhenUnconnected=off
  EgrCoolerTempOut : Outport  Port=19  VectorParamsAs1DForOutWhenUnconnected=off
  EO HC : Outport  Port=20  VectorParamsAs1DForOutWhenUnconnected=off
  EO CO : Outport  Port=21  VectorParamsAs1DForOutWhenUnconnected=off
  EO NOx : Outport  Port=22  VectorParamsAs1DForOutWhenUnconnected=off
  EO CO2 : Outport  Port=23  VectorParamsAs1DForOutWhenUnconnected=off
  Iat : Outport  Port=24  VectorParamsAs1DForOutWhenUnconnected=off
  Ect : Outport  Port=25  VectorParamsAs1DForOutWhenUnconnected=off
  EgrVlvDeltaPrs : Outport  Port=26  VectorParamsAs1DForOutWhenUnconnected=off
  EgrVlvInTemp : Outport  Port=27  VectorParamsAs1DForOutWhenUnconnected=off
  wires:
  EgrVlvAreaPct/1 -> EGR/1(EgrVlvAreaPct)
  EGR/1(EgrInfo) -> [EgrInfo]
  EngSpd/1 -> CI Core Engine/3
  [AmbTemp] -> Intercooler/1
  [AmbTemp] -> Environment Exhaust/2
  [AmbPrs] -> Environment Exhaust/1
  Environment Intake/1 -> [EnvInfo]
  AmbPrs/1 -> [AmbPrs]
  AmbTemp/1 -> [AmbTemp]
  Turbine/1 -> [TurbInfo]
  Boost Drive Shaft/1 -> [TurboShaftInfo]
  Exhaust Manifold/1 -> [ExhInfo]
  CI Core Engine/1 -> [CoreEngInfo]
  Intake Manifold/1 -> [IntkInfo]
  Compressor/1 -> [CompInfo]
  CI Core Engine/2 -> EngTrq/1  "EngTrq"
  Intercooler/1 -> [IntercoolerInfo]
  Air Filter/1 -> Terminator5/1
  Air Intake System/1 -> [AirIntkVolInfo]
  Exhaust System Volume/1 -> [TurbOutVolInfo]
  Exhaust Back Pressure/1 -> [ExhOutFlwInfo]
  Environment Exhaust/1 -> Terminator1/1
  [AmbPrs] -> Environment Intake/1
  [AmbTemp] -> Environment Intake/2
  [EnvInfo] -> Subsystem/1(EnvInfo)
  [IntkInfo] -> Subsystem/2(IntkInfo)
  [ExhInfo] -> Subsystem/3(ExhInfo)
  [CoreEngInfo] -> Subsystem/4(CoreEngInfo)
  [CompInfo] -> Subsystem/5(CompInfo)
  [TurbInfo] -> Subsystem/6(TurbInfo)
  [IntercoolerInfo] -> Subsystem/7(IntercoolerInfo)
  [TurboShaftInfo] -> Subsystem/8(TurboShaftInfo)
  Subsystem/1(IntkPortFlw) -> IntkPortFlw/1
  Subsystem/5(ExhMap) -> ExhMap/1
  Subsystem/4(Mat) -> Mat/1
  Subsystem/3(Map) -> Map/1
  Subsystem/6(ExhMat) -> ExhMat/1
  Subsystem/7(FuelFlw) -> FuelFlw/1
  Subsystem/9(Afr) -> Afr/1
  Subsystem/2(NormAirChrg) -> NormAirChrg/1
  Subsystem/10(TurboSpd) -> TurboSpd/1
  Subsystem/11(TurbPrsRatio) -> TurbPrsRatio/1
  Subsystem/12(CompPrsRatio) -> CompPrsRatio/1
  Subsystem/13(TurbTempOut) -> TurbTempOut/1
  Subsystem/14(CompTempOut) -> CompTempOut/1
  Subsystem/15(IntercoolerTempOut) -> IntercoolerTempOut/1
  [TurbOutVolInfo] -> Subsystem/10(TurbOutVolInfo)
  [EgrInfo] -> Subsystem/9(EgrInfo)
  Subsystem/16(EgrPct) -> EgrPct/1
  Subsystem/17(EgrMassFlwRate) -> EgrMassFlwRate/1
  Subsystem/18(EgrCoolerTempOut) -> EgrCoolerTempOut/1
  FuelMainSoi/1 -> CI Core Engine/2
  [ExhOutFlwInfo] -> Subsystem/11(ExhOutFlwInfo)
  Subsystem/19(EO HC) -> EO HC/1
  Subsystem/20(EO CO) -> EO CO/1
  Subsystem/21(EO NOx) -> EO NOx/1
  Subsystem/22(EO CO2) -> EO CO2/1
  InjPw/1 -> Fuel System/1(InjPw)
  Fuel System/1(FuelMassPerInj) -> CI Core Engine/1
  TurboRackPos/1 -> Turbine/1
  Subsystem/24(Ect) -> Ect/1
  [UndHdTemp] -> Engine Coolant Temperature/3(UndHdTemp)
  [IntkInfo] -> Engine Coolant Temperature/2(IntkInfo)
  [UndHdFlwVel] -> Engine Coolant Temperature/4(UndHdFlwVel)
  [CoreEngInfo] -> Engine Coolant Temperature/1(CoreEngInfo)
  UndHdFlwVel/1 -> [UndHdFlwVel]
  UndHdTemp/1 -> [UndHdTemp]
  [UndHdTemp] -> Intake Manifold/2
  [UndHdFlwVel] -> Intake Manifold/1
  Engine Coolant Temperature/1(EngThermInfo) -> [EngThermInfo]
  Engine Coolant Temperature/2(Ect) -> CI Core Engine/5
  [EngThermInfo] -> Subsystem/12(EngThermInfo)
  Subsystem/25(EgrVlvDeltaPrs) -> EgrVlvDeltaPrs/1
  Subsystem/26(EgrVlvInTemp) -> EgrVlvInTemp/1
  [AirIntkVolInfo] -> Subsystem/13(AirIntkVolInfo)
  Subsystem/23(Iat) -> Iat/1
  FuelPrs/1 -> CI Core Engine/4
  Subsystem/8(FuelVolFlw) -> FuelVolFlw/1
  connections:
  Exhaust Manifold/LConn1 -- CI Core Engine/RConn1
  Intake Manifold/LConn1 -- EGR/RConn1
  Exhaust Manifold/RConn1 -- EGR/LConn1
  Compressor/LConn1 -- Intercooler/LConn1
  Compressor/LConn2 -- Boost Drive Shaft/LConn1
  Turbine/RConn1 -- Boost Drive Shaft/RConn1
  Exhaust Back Pressure/LConn1 -- Exhaust System Volume/RConn1
  CI Core Engine/LConn1 -- Intake Manifold/RConn1
  Environment Intake/RConn1 -- Air Filter/LConn1
  Environment Exhaust/RConn1 -- Exhaust Back Pressure/RConn1
  Compressor/RConn1 -- Air Intake System/RConn1
  Intercooler/RConn1 -- Intake Manifold/LConn2
  Turbine/LConn1 -- Exhaust Manifold/RConn2
  Exhaust System Volume/LConn1 -- Turbine/LConn2
  Air Filter/RConn1 -- Air Intake System/LConn1
